simulink model "AdaptiveMPC_Simulation"  (R2020a)
settings: Solver=ode45  StartTime=0  StopTime=150  MaxStep=0.5*Ts  RelTol=1e-3  EnableMultiTasking=on
values from neighbouring files (symbols this model uses):
  Ts = 0.5    [MPC_controller_parameters.m]
  u0 = [op_report.Inputs(1).u;op_report.Inputs(2).u;op_report.Inputs(3).u]    [MPC_controller_parameters.m]
  x0 = [op_report.States(1).x;op_report.States(2).x]    [MPC_controller_parameters.m]
  y0 = [op_report.Outputs(1).y;op_report.Outputs(2).y]    [MPC_controller_parameters.m]
libraries: mpclib x1, dspstat3 x1, slident x1, simulink x1
settings Model: Creator=The MathWorks, Inc.  LastModifiedBy=Mirza
settings DataIOCC: ExternalInput=ExtIn  InitialState=[311.267; 8.5695]  SaveFormat=Structure  SaveOutput=off  SignalLogging=off  DSMLogging=off  SaveTime=off  ReturnWorkspaceOutputs=off  SignalLoggingName=logsOut
settings OptimizationCC: BooleanDataType=off  DefaultParameterBehavior=Inlined  InlineInvariantSignals=on  BufferReuse=off  ExpressionDepthLimit=2147483647  InitFltsAndDblsToZero=on  LifeSpan=inf
settings DebuggingCC: SaveWithParameterizedLinksMsg=none  UnderspecifiedInitializationDetection=Classic  MergeDetectMultiDrivingBlocksExec=none  CheckExecutionContextPreStartOutputMsg=on  CheckExecutionContextRuntimeOutputMsg=on  SignalResolutionControl=TryResolveAllWithWarning  MultiTaskDSMMsg=warning  MultiTaskCondExecSysMsg=none  StateNameClashWarn=warning  SFUnexpectedBacktrackingDiag=warning  SFNoUnconditionalDefaultTransitionDiag=warning  SFExecutionAtInitializationDiag=none  ArithmeticOperatorsInVariantConditions=warning
settings HardwareCC: ProdBitPerPointer=32  ProdBitPerSizeT=32  ProdBitPerPtrDiffT=32  ProdLargestAtomicFloat=None  ProdIntDivRoundTo=Undefined  ProdEndianess=Unspecified  ProdWordSize=32  ProdHWDeviceType=32-bit Generic  TargetUnknown=on
settings ModelReferenceCC: PropagateSignalLabelsOutOfModel=off
settings SFSimCC: SimUseLocalCustomCode=off  CustomCodeUndefinedFunction=UseInterfaceOnly
settings RTWCC: RTWUseLocalCustomCode=off
settings CodeAppCC: StateflowObjectComments=on
settings GRTTargetCC: TargetFcnLib=ansi_tfl_tmw.mat  TargetLangStandard=C89/C90 (ANSI)  CombineOutputUpdateFcns=off  GRTInterface=on
settings ConfigComp: CovMetricSettings=dw  CovHtmlReporting=on  CovSaveCumulativeToWorkspaceVar=on  CovSaveSingleToWorkspaceVar=on  CovExternalEMLEnable=off  CovSFcnEnable=off

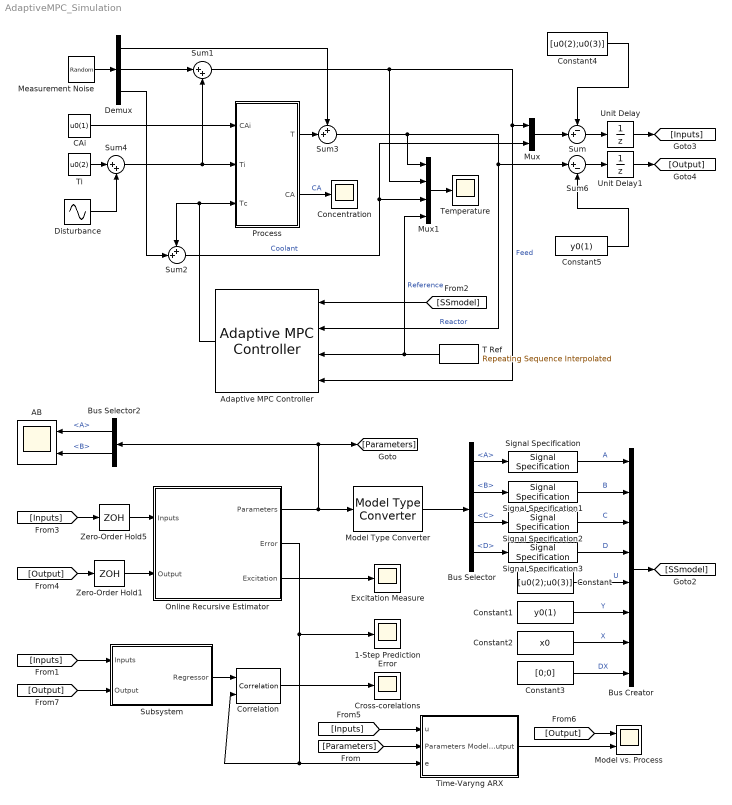
== system AdaptiveMPC_Simulation ==
  1-Step Prediction Error : Scope
  AB : Scope  NumInputPorts=2
  Adaptive MPC Controller : mpclib/Adaptive MPC Controller  SCDEnableBlockLinearizationSpecification=on  mpcobj=mpcobj  enable_value=0  updateMPCinCallerWorkspace=on  md_inport=on  mv_inport=off  uref_inport=off  return_cost=off  return_mvseq=off  return_qpstatus=off  return_xseq=off  return_state=off  return_ovseq=off  state_inport=off  isltv_plant=off  umin_inport=off  umax_inport=off  ymin_inport=off  ymax_inport=off  cc_inport=off  ywt_inport=off  uwt_inport=off  duwt_inport=off  rhoeps_inport=off  pm_inport=off  MaximumP=10  HorizonChoice=FixedHorizon  BlockDataType=double  SampleTimeInherited=off  switch_inport=off
  Bus Creator : BusCreator  Inputs=8
  Bus Selector : BusSelector  OutputSignals=A,B,C,D
  Bus Selector2 : BusSelector  OutputSignals=A,B
  CAi : Constant  Value=u0(1)
  Concentration : Scope
  Constant : Constant  Value=[u0(2);u0(3)]  VectorParams1D=off
  Constant1 : Constant  Value=y0(1)  VectorParams1D=off
  Constant2 : Constant  Value=x0  VectorParams1D=off
  Constant3 : Constant  Value=[0;0]  VectorParams1D=off
  Constant4 : Constant  Value=[u0(2);u0(3)]
  Constant5 : Constant  Value=y0(1)
  Correlation : dspstat3/Correlation  domain=Time  roundingMode=Floor  overflowMode=off  outputDataTypeStr=Inherit: Same as accumulator  outputMin=[]  outputMax=[]  outputLastDataTypeStr=Inherit: Same as accumulator
      settings: SourceProductBaseCode=DS
  Cross-corelations : Scope
  Demux : Demux  Outputs=3
  Disturbance : Sin  Amplitude=5  Frequency=0.05  SampleTime=0
  Excitation Measure : Scope
  Measurement Noise : RandomNumber  Mean=[0 0 0]  Variance=0.001*[1 1 1]  Seed=12345  SampleTime=Ts/5
  Model Type Converter : slident/Estimators/Model Type Converter  InputModelType=ARX
      settings: SourceProductBaseCode=ID
  Model vs. Process : Scope  NumInputPorts=2
  Mux : Mux  Inputs=2
  Mux1 : Mux
  Online Recursive Estimator : Subsystem  mask{ModelStructure=ARX, A0=2, B0=[2 2], F0=2, C0=2, D0=2, d=[0 0], P0=10, History=Infinitna, WindowLength=100, EstimationMethod=Kalmanov filter, Lambda=1 - 5e-3, ProcessNoiseCovariance=1, Tolerance=0.0001, AddEnablePort=off, EstimationError=on, ExcitationMeasure=on, SampleTime=0.5}
      mask prompts: ModelStructure "Izbor modela:"; A0 "Broj parametara u A(q) (na):"; B0 "Broj parametara u B(q) (nb):"; F0 "Broj parametara u F(q) (nf):"; C0 "Broj parametara u C(q) (nc):"; D0 "Broj parametara u D(q) (nd):"; d "Kasnjenje ulaza (nk):"; P0 "Matrica kovarijanse parametara:"; History "Historija:"; WindowLength "Sirina prozora:"; EstimationMethod "Metod estimacije:"; Lambda "Faktor iscezavanja:"; ProcessNoiseCovariance "Kovarijansa procesnog suma:"; Tolerance "Toleranca:"; AddEnablePort "Enable port"; EstimationError "Greska estimacije:"; ExcitationMeasure "Mjera pobude:"; SampleTime "Period uzorkovanja:"
      mask TypeOptions ModelStructure: ARX | ARMAX | BJ | OE
      mask Callback ModelStructure:
      | maskStr = get_param(gcb, 'ModelStructure');
      | maskStr1 = get_param(gcb, 'History');
      | maskStr2 = get_param(gcb, 'EstimationMethod');
      | 
      | if strcmp(maskStr, 'ARX') && strcmp(maskStr1, 'Infinitna') && strcmp(maskStr2, 'Faktor iscezavanja') ,
      |     set_param(gcb, 'MaskVisibilities', {'on';'on';'on';'off';'off';'off';'on';'on';'on';'off';'on';'on';'off';'off';'on';'on';'on';'on'}),
      | elseif strcmp(maskStr, 'ARX') && strcmp(maskStr1, 'Infinitna') && strcmp(maskStr2, 'BFGS') ,
      |     set_param(gcb, 'MaskVisibilities', {'on';'on';'on';'off';'off';'off';'on';'on';'on';'on';'on';'off';'off';'on';'on';'on';'on';'on'}),
      | elseif strcmp(maskStr, 'ARX') && strcmp(maskStr1, 'Infinitna') && strcmp(maskStr2, 'Kalmanov filter') ,
      |     set_param(gcb, 'MaskVisibilities', {'on';'on';'on';'off';'off';'off';'on';'on';'on';'off';'on';'off';'on';'off';'on';'on';'on';'on'}),
      | elseif strcmp(maskStr, 'ARX') && strcmp(maskStr1, 'Finitna') && strcmp(maskStr2, 'Faktor iscezavanja') ,
      |     set_param(gcb, 'MaskVisibilities', {'on';'on';'on';'off';'off';'off';'on';'on';'on';'on';'on';'off';'off';'off';'on';'on';'on';'on'}),
      | elseif strcmp(maskStr, 'ARX') && strcmp(maskStr1, 'Finitna') && strcmp(maskStr2, 'BFGS') ,
      |     set_param(gcb, 'MaskVisibilities', {'on';'on';'on';'off';'off';'off';'on';'on';'on';'on';'on';'off';'off';'on';'on';'on';'on';'on'}),
      | elseif strcmp(maskStr, 'ARX') && strcmp(maskStr1, 'Finitna') && strcmp(maskStr2, 'Kalmanov filter') ,
      |     set_param(gcb, 'MaskVisibilities', {'on';'on';'on';'off';'off';'off';'on';'on';'on';'on';'on';'off';'off';'off';'on';'on';'on';'on'}),
      | elseif strcmp(maskStr, 'ARMAX') && strcmp(maskStr1, 'Infinitna') && strcmp(maskStr2, 'Faktor iscezavanja') ,
      |     set_param(gcb, 'MaskVisibilities', {'on';'on';'on';'off';'on';'off';'on';'on';'on';'off';'on';'on';'off';'off';'on';'on';'on';'on'}),
      | elseif strcmp(maskStr, 'ARMAX') && strcmp(maskStr1, 'Infinitna') && strcmp(maskStr2, 'BFGS') ,
      |     set_param(gcb, 'MaskVisibilities', {'on';'on';'on';'off';'on';'off';'on';'on';'on';'on';'on';'off';'off';'on';'on';'on';'on';'on'}),
      | elseif strcmp(maskStr, 'ARMAX') && strcmp(maskStr1, 'Infinitna') && strcmp(maskStr2, 'Kalmanov filter') ,
      |     set_param(gcb, 'MaskVisibilities', {'on';'on';'on';'off';'on';'off';'on';'on';'on';'off';'on';'off';'on';'off';'on';'on';'on';'on'}),
      | elseif strcmp(maskStr, 'ARMAX') && strcmp(maskStr1, 'Finitna') && strcmp(maskStr2, 'Faktor iscezavanja') ,
      |     set_param(gcb, 'MaskVisibilities', {'on';'on';'on';'off';'on';'off';'on';'on';'on';'on';'on';'off';'off';'off';'on';'on';'on';'on'}),
      | elseif strcmp(maskStr, 'ARMAX') && strcmp(maskStr1, 'Finitna') && strcmp(maskStr2, 'BFGS') ,
      |     set_param(gcb, 'MaskVisibilities', {'on';'on';'on';'off';'on';'off';'on';'on';'on';'on';'on';'off';'off';'on';'on';'on';'on';'on'}),
      | elseif strcmp(maskStr, 'ARMAX') && strcmp(maskStr1, 'Finitna') && strcmp(maskStr2, 'Kalmanov filter') ,
      |     set_param(gcb, 'MaskVisibilities', {'on';'on';'on';'off';'on';'off';'on';'on';'on';'on';'on';'off';'off';'off';'on';'on';'on';'on'}),
      | elseif strcmp(maskStr, 'BJ') && strcmp(maskStr1, 'Infinitna') && strcmp(maskStr2, 'Faktor iscezavanja') ,
      |     set_param(gcb, 'MaskVisibilities', {'on';'off';'on';'on';'on';'on';'on';'on';'on';'off';'on';'on';'off';'off';'on';'on';'on';'on'}),
      | elseif strcmp(maskStr, 'BJ') && strcmp(maskStr1, 'Infinitna') && strcmp(maskStr2, 'BFGS') ,
      |     set_param(gcb, 'MaskVisibilities', {'on';'off';'on';'on';'on';'on';'on';'on';'on';'on';'on';'off';'off';'on';'on';'on';'on';'on'}),
      | elseif strcmp(maskStr, 'BJ') && strcmp(maskStr1, 'Infinitna') && strcmp(maskStr2, 'Kalmanov filter') ,
      |     set_param(gcb, 'MaskVisibilities', {'on';'off';'on';'on';'on';'on';'on';'on';'on';'off';'on';'off';'on';'off';'on';'on';'on';'on'}),
      | elseif strcmp(maskStr, 'BJ') && strcmp(maskStr1, 'Finitna') && strcmp(maskStr2, 'Faktor iscezavanja') ,
      |     set_param(gcb, 'MaskVisibilities', {'on';'off';'on';'on';'on';'on';'on';'on';'on';'on';'on';'off';'off';'off';'on';'on';'on';'on'}),
      | elseif strcmp(maskStr, 'BJ') && strcmp(maskStr1, 'Finitna') && strcmp(maskStr2, 'BFGS') ,
      |     set_param(gcb, 'MaskVisibilities', {'on';'off';'on';'on';'on';'on';'on';'on';'on';'on';'on';'off';'off';'on';'on';'on';'on';'on'}),
      | elseif strcmp(maskStr, 'BJ') && strcmp(maskStr1, 'Finitna') && strcmp(maskStr2, 'Kalmanov filter') ,
      |     set_param(gcb, 'MaskVisibilities', {'on';'off';'on';'on';'on';'on';'on';'on';'on';'on';'on';'off';'off';'off';'on';'on';'on';'on'}),
      | elseif strcmp(maskStr, 'OE') && strcmp(maskStr1, 'Infinitna') && strcmp(maskStr2, 'Faktor iscezavanja') ,
      |     set_param(gcb, 'MaskVisibilities', {'on';'off';'on';'on';'off';'off';'on';'on';'on';'off';'on';'on';'off';'off';'on';'on';'on';'on'}),
      | elseif strcmp(maskStr, 'OE') && strcmp(maskStr1, 'Infinitna') && strcmp(maskStr2, 'BFGS') ,
      |     set_param(gcb, 'MaskVisibilities', {'on';'off';'on';'on';'off';'off';'on';'on';'on';'on';'on';'off';'off';'on';'on';'on';'on';'on'}),
      | elseif strcmp(maskStr, 'OE') && strcmp(maskStr1, 'Infinitna') && strcmp(maskStr2, 'Kalmanov filter') ,
      |     set_param(gcb, 'MaskVisibilities', {'on';'off';'on';'on';'off';'off';'on';'on';'on';'off';'on';'off';'on';'off';'on';'on';'on';'on'}),
      | elseif strcmp(maskStr, 'OE') && strcmp(maskStr1, 'Finitna') && strcmp(maskStr2, 'Faktor iscezavanja') ,
      |     set_param(gcb, 'MaskVisibilities', {'on';'off';'on';'on';'off';'off';'on';'on';'on';'on';'on';'off';'off';'off';'on';'on';'on';'on'}),
      | elseif strcmp(maskStr, 'OE') && strcmp(maskStr1, 'Finitna') && strcmp(maskStr2, 'BFGS') ,
      |     set_param(gcb, 'MaskVisibilities', {'on';'off';'on';'on';'off';'off';'on';'on';'on';'on';'on';'off';'off';'on';'on';'on';'on';'on'}),
      | elseif strcmp(maskStr, 'OE') && strcmp(maskStr1, 'Finitna') && strcmp(maskStr2, 'Kalmanov filter') ,
      |     set_param(gcb, 'MaskVisibilities', {'on';'off';'on';'on';'off';'off';'on';'on';'on';'on';'on';'off';'off';'off';'on';'on';'on';'on'}),
      | end
      mask TypeOptions History: Infinitna | Finitna
      mask Callback History:
      | maskStr = get_param(gcb, 'ModelStructure');
      | maskStr1 = get_param(gcb, 'History');
      | maskStr2 = get_param(gcb, 'EstimationMethod');
      | 
      | if strcmp(maskStr, 'ARX') && strcmp(maskStr1, 'Infinitna') && strcmp(maskStr2, 'Faktor iscezavanja') ,
      |     set_param(gcb, 'MaskVisibilities', {'on';'on';'on';'off';'off';'off';'on';'on';'on';'off';'on';'on';'off';'off';'on';'on';'on';'on'}),
      | elseif strcmp(maskStr, 'ARX') && strcmp(maskStr1, 'Infinitna') && strcmp(maskStr2, 'BFGS') ,
      |     set_param(gcb, 'MaskVisibilities', {'on';'on';'on';'off';'off';'off';'on';'on';'on';'on';'on';'off';'off';'on';'on';'on';'on';'on'}),
      | elseif strcmp(maskStr, 'ARX') && strcmp(maskStr1, 'Infinitna') && strcmp(maskStr2, 'Kalmanov filter') ,
      |     set_param(gcb, 'MaskVisibilities', {'on';'on';'on';'off';'off';'off';'on';'on';'on';'off';'on';'off';'on';'off';'on';'on';'on';'on'}),
      | elseif strcmp(maskStr, 'ARX') && strcmp(maskStr1, 'Finitna') && strcmp(maskStr2, 'Faktor iscezavanja') ,
      |     set_param(gcb, 'MaskVisibilities', {'on';'on';'on';'off';'off';'off';'on';'on';'on';'on';'on';'off';'off';'off';'on';'on';'on';'on'}),
      | elseif strcmp(maskStr, 'ARX') && strcmp(maskStr1, 'Finitna') && strcmp(maskStr2, 'BFGS') ,
      |     set_param(gcb, 'MaskVisibilities', {'on';'on';'on';'off';'off';'off';'on';'on';'on';'on';'on';'off';'off';'on';'on';'on';'on';'on'}),
      | elseif strcmp(maskStr, 'ARX') && strcmp(maskStr1, 'Finitna') && strcmp(maskStr2, 'Kalmanov filter') ,
      |     set_param(gcb, 'MaskVisibilities', {'on';'on';'on';'off';'off';'off';'on';'on';'on';'on';'on';'off';'off';'off';'on';'on';'on';'on'}),
      | elseif strcmp(maskStr, 'ARMAX') && strcmp(maskStr1, 'Infinitna') && strcmp(maskStr2, 'Faktor iscezavanja') ,
      |     set_param(gcb, 'MaskVisibilities', {'on';'on';'on';'off';'on';'off';'on';'on';'on';'off';'on';'on';'off';'off';'on';'on';'on';'on'}),
      | elseif strcmp(maskStr, 'ARMAX') && strcmp(maskStr1, 'Infinitna') && strcmp(maskStr2, 'BFGS') ,
      |     set_param(gcb, 'MaskVisibilities', {'on';'on';'on';'off';'on';'off';'on';'on';'on';'on';'on';'off';'off';'on';'on';'on';'on';'on'}),
      | elseif strcmp(maskStr, 'ARMAX') && strcmp(maskStr1, 'Infinitna') && strcmp(maskStr2, 'Kalmanov filter') ,
      |     set_param(gcb, 'MaskVisibilities', {'on';'on';'on';'off';'on';'off';'on';'on';'on';'off';'on';'off';'on';'off';'on';'on';'on';'on'}),
      | elseif strcmp(maskStr, 'ARMAX') && strcmp(maskStr1, 'Finitna') && strcmp(maskStr2, 'Faktor iscezavanja') ,
      |     set_param(gcb, 'MaskVisibilities', {'on';'on';'on';'off';'on';'off';'on';'on';'on';'on';'on';'off';'off';'off';'on';'on';'on';'on'}),
      | elseif strcmp(maskStr, 'ARMAX') && strcmp(maskStr1, 'Finitna') && strcmp(maskStr2, 'BFGS') ,
      |     set_param(gcb, 'MaskVisibilities', {'on';'on';'on';'off';'on';'off';'on';'on';'on';'on';'on';'off';'off';'on';'on';'on';'on';'on'}),
      | elseif strcmp(maskStr, 'ARMAX') && strcmp(maskStr1, 'Finitna') && strcmp(maskStr2, 'Kalmanov filter') ,
      |     set_param(gcb, 'MaskVisibilities', {'on';'on';'on';'off';'on';'off';'on';'on';'on';'on';'on';'off';'off';'off';'on';'on';'on';'on'}),
      | elseif strcmp(maskStr, 'BJ') && strcmp(maskStr1, 'Infinitna') && strcmp(maskStr2, 'Faktor iscezavanja') ,
      |     set_param(gcb, 'MaskVisibilities', {'on';'off';'on';'on';'on';'on';'on';'on';'on';'off';'on';'on';'off';'off';'on';'on';'on';'on'}),
      | elseif strcmp(maskStr, 'BJ') && strcmp(maskStr1, 'Infinitna') && strcmp(maskStr2, 'BFGS') ,
      |     set_param(gcb, 'MaskVisibilities', {'on';'off';'on';'on';'on';'on';'on';'on';'on';'on';'on';'off';'off';'on';'on';'on';'on';'on'}),
      | elseif strcmp(maskStr, 'BJ') && strcmp(maskStr1, 'Infinitna') && strcmp(maskStr2, 'Kalmanov filter') ,
      |     set_param(gcb, 'MaskVisibilities', {'on';'off';'on';'on';'on';'on';'on';'on';'on';'off';'on';'off';'on';'off';'on';'on';'on';'on'}),
      | elseif strcmp(maskStr, 'BJ') && strcmp(maskStr1, 'Finitna') && strcmp(maskStr2, 'Faktor iscezavanja') ,
      |     set_param(gcb, 'MaskVisibilities', {'on';'off';'on';'on';'on';'on';'on';'on';'on';'on';'on';'off';'off';'off';'on';'on';'on';'on'}),
      | elseif strcmp(maskStr, 'BJ') && strcmp(maskStr1, 'Finitna') && strcmp(maskStr2, 'BFGS') ,
      |     set_param(gcb, 'MaskVisibilities', {'on';'off';'on';'on';'on';'on';'on';'on';'on';'on';'on';'off';'off';'on';'on';'on';'on';'on'}),
      | elseif strcmp(maskStr, 'BJ') && strcmp(maskStr1, 'Finitna') && strcmp(maskStr2, 'Kalmanov filter') ,
      |     set_param(gcb, 'MaskVisibilities', {'on';'off';'on';'on';'on';'on';'on';'on';'on';'on';'on';'off';'off';'off';'on';'on';'on';'on'}),
      | elseif strcmp(maskStr, 'OE') && strcmp(maskStr1, 'Infinitna') && strcmp(maskStr2, 'Faktor iscezavanja') ,
      |     set_param(gcb, 'MaskVisibilities', {'on';'off';'on';'on';'off';'off';'on';'on';'on';'off';'on';'on';'off';'off';'on';'on';'on';'on'}),
      | elseif strcmp(maskStr, 'OE') && strcmp(maskStr1, 'Infinitna') && strcmp(maskStr2, 'BFGS') ,
      |     set_param(gcb, 'MaskVisibilities', {'on';'off';'on';'on';'off';'off';'on';'on';'on';'on';'on';'off';'off';'on';'on';'on';'on';'on'}),
      | elseif strcmp(maskStr, 'OE') && strcmp(maskStr1, 'Infinitna') && strcmp(maskStr2, 'Kalmanov filter') ,
      |     set_param(gcb, 'MaskVisibilities', {'on';'off';'on';'on';'off';'off';'on';'on';'on';'off';'on';'off';'on';'off';'on';'on';'on';'on'}),
      | elseif strcmp(maskStr, 'OE') && strcmp(maskStr1, 'Finitna') && strcmp(maskStr2, 'Faktor iscezavanja') ,
      |     set_param(gcb, 'MaskVisibilities', {'on';'off';'on';'on';'off';'off';'on';'on';'on';'on';'on';'off';'off';'off';'on';'on';'on';'on'}),
      | elseif strcmp(maskStr, 'OE') && strcmp(maskStr1, 'Finitna') && strcmp(maskStr2, 'BFGS') ,
      |     set_param(gcb, 'MaskVisibilities', {'on';'off';'on';'on';'off';'off';'on';'on';'on';'on';'on';'off';'off';'on';'on';'on';'on';'on'}),
      | elseif strcmp(maskStr, 'OE') && strcmp(maskStr1, 'Finitna') && strcmp(maskStr2, 'Kalmanov filter') ,
      |     set_param(gcb, 'MaskVisibilities', {'on';'off';'on';'on';'off';'off';'on';'on';'on';'on';'on';'off';'off';'off';'on';'on';'on';'on'}),
      | end
      mask TypeOptions EstimationMethod: Faktor iscezavanja | BFGS | Kalmanov filter
      mask Callback EstimationMethod:
      | maskStr = get_param(gcb, 'ModelStructure');
      | maskStr1 = get_param(gcb, 'History');
      | maskStr2 = get_param(gcb, 'EstimationMethod');
      | 
      | if strcmp(maskStr, 'ARX') && strcmp(maskStr1, 'Infinitna') && strcmp(maskStr2, 'Faktor iscezavanja') ,
      |     set_param(gcb, 'MaskVisibilities', {'on';'on';'on';'off';'off';'off';'on';'on';'on';'off';'on';'on';'off';'off';'on';'on';'on';'on'}),
      | elseif strcmp(maskStr, 'ARX') && strcmp(maskStr1, 'Infinitna') && strcmp(maskStr2, 'BFGS') ,
      |     set_param(gcb, 'MaskVisibilities', {'on';'on';'on';'off';'off';'off';'on';'on';'on';'on';'on';'off';'off';'on';'on';'on';'on';'on'}),
      | elseif strcmp(maskStr, 'ARX') && strcmp(maskStr1, 'Infinitna') && strcmp(maskStr2, 'Kalmanov filter') ,
      |     set_param(gcb, 'MaskVisibilities', {'on';'on';'on';'off';'off';'off';'on';'on';'on';'off';'on';'off';'on';'off';'on';'on';'on';'on'}),
      | elseif strcmp(maskStr, 'ARX') && strcmp(maskStr1, 'Finitna') && strcmp(maskStr2, 'Faktor iscezavanja') ,
      |     set_param(gcb, 'MaskVisibilities', {'on';'on';'on';'off';'off';'off';'on';'on';'on';'on';'on';'off';'off';'off';'on';'on';'on';'on'}),
      | elseif strcmp(maskStr, 'ARX') && strcmp(maskStr1, 'Finitna') && strcmp(maskStr2, 'BFGS') ,
      |     set_param(gcb, 'MaskVisibilities', {'on';'on';'on';'off';'off';'off';'on';'on';'on';'on';'on';'off';'off';'on';'on';'on';'on';'on'}),
      | elseif strcmp(maskStr, 'ARX') && strcmp(maskStr1, 'Finitna') && strcmp(maskStr2, 'Kalmanov filter') ,
      |     set_param(gcb, 'MaskVisibilities', {'on';'on';'on';'off';'off';'off';'on';'on';'on';'on';'on';'off';'off';'off';'on';'on';'on';'on'}),
      | elseif strcmp(maskStr, 'ARMAX') && strcmp(maskStr1, 'Infinitna') && strcmp(maskStr2, 'Faktor iscezavanja') ,
      |     set_param(gcb, 'MaskVisibilities', {'on';'on';'on';'off';'on';'off';'on';'on';'on';'off';'on';'on';'off';'off';'on';'on';'on';'on'}),
      | elseif strcmp(maskStr, 'ARMAX') && strcmp(maskStr1, 'Infinitna') && strcmp(maskStr2, 'BFGS') ,
      |     set_param(gcb, 'MaskVisibilities', {'on';'on';'on';'off';'on';'off';'on';'on';'on';'on';'on';'off';'off';'on';'on';'on';'on';'on'}),
      | elseif strcmp(maskStr, 'ARMAX') && strcmp(maskStr1, 'Infinitna') && strcmp(maskStr2, 'Kalmanov filter') ,
      |     set_param(gcb, 'MaskVisibilities', {'on';'on';'on';'off';'on';'off';'on';'on';'on';'off';'on';'off';'on';'off';'on';'on';'on';'on'}),
      | elseif strcmp(maskStr, 'ARMAX') && strcmp(maskStr1, 'Finitna') && strcmp(maskStr2, 'Faktor iscezavanja') ,
      |     set_param(gcb, 'MaskVisibilities', {'on';'on';'on';'off';'on';'off';'on';'on';'on';'on';'on';'off';'off';'off';'on';'on';'on';'on'}),
      | elseif strcmp(maskStr, 'ARMAX') && strcmp(maskStr1, 'Finitna') && strcmp(maskStr2, 'BFGS') ,
      |     set_param(gcb, 'MaskVisibilities', {'on';'on';'on';'off';'on';'off';'on';'on';'on';'on';'on';'off';'off';'on';'on';'on';'on';'on'}),
      | elseif strcmp(maskStr, 'ARMAX') && strcmp(maskStr1, 'Finitna') && strcmp(maskStr2, 'Kalmanov filter') ,
      |     set_param(gcb, 'MaskVisibilities', {'on';'on';'on';'off';'on';'off';'on';'on';'on';'on';'on';'off';'off';'off';'on';'on';'on';'on'}),
      | elseif strcmp(maskStr, 'BJ') && strcmp(maskStr1, 'Infinitna') && strcmp(maskStr2, 'Faktor iscezavanja') ,
      |     set_param(gcb, 'MaskVisibilities', {'on';'off';'on';'on';'on';'on';'on';'on';'on';'off';'on';'on';'off';'off';'on';'on';'on';'on'}),
      | elseif strcmp(maskStr, 'BJ') && strcmp(maskStr1, 'Infinitna') && strcmp(maskStr2, 'BFGS') ,
      |     set_param(gcb, 'MaskVisibilities', {'on';'off';'on';'on';'on';'on';'on';'on';'on';'on';'on';'off';'off';'on';'on';'on';'on';'on'}),
      | elseif strcmp(maskStr, 'BJ') && strcmp(maskStr1, 'Infinitna') && strcmp(maskStr2, 'Kalmanov filter') ,
      |     set_param(gcb, 'MaskVisibilities', {'on';'off';'on';'on';'on';'on';'on';'on';'on';'off';'on';'off';'on';'off';'on';'on';'on';'on'}),
      | elseif strcmp(maskStr, 'BJ') && strcmp(maskStr1, 'Finitna') && strcmp(maskStr2, 'Faktor iscezavanja') ,
      |     set_param(gcb, 'MaskVisibilities', {'on';'off';'on';'on';'on';'on';'on';'on';'on';'on';'on';'off';'off';'off';'on';'on';'on';'on'}),
      | elseif strcmp(maskStr, 'BJ') && strcmp(maskStr1, 'Finitna') && strcmp(maskStr2, 'BFGS') ,
      |     set_param(gcb, 'MaskVisibilities', {'on';'off';'on';'on';'on';'on';'on';'on';'on';'on';'on';'off';'off';'on';'on';'on';'on';'on'}),
      | elseif strcmp(maskStr, 'BJ') && strcmp(maskStr1, 'Finitna') && strcmp(maskStr2, 'Kalmanov filter') ,
      |     set_param(gcb, 'MaskVisibilities', {'on';'off';'on';'on';'on';'on';'on';'on';'on';'on';'on';'off';'off';'off';'on';'on';'on';'on'}),
      | elseif strcmp(maskStr, 'OE') && strcmp(maskStr1, 'Infinitna') && strcmp(maskStr2, 'Faktor iscezavanja') ,
      |     set_param(gcb, 'MaskVisibilities', {'on';'off';'on';'on';'off';'off';'on';'on';'on';'off';'on';'on';'off';'off';'on';'on';'on';'on'}),
      | elseif strcmp(maskStr, 'OE') && strcmp(maskStr1, 'Infinitna') && strcmp(maskStr2, 'BFGS') ,
      |     set_param(gcb, 'MaskVisibilities', {'on';'off';'on';'on';'off';'off';'on';'on';'on';'on';'on';'off';'off';'on';'on';'on';'on';'on'}),
      | elseif strcmp(maskStr, 'OE') && strcmp(maskStr1, 'Infinitna') && strcmp(maskStr2, 'Kalmanov filter') ,
      |     set_param(gcb, 'MaskVisibilities', {'on';'off';'on';'on';'off';'off';'on';'on';'on';'off';'on';'off';'on';'off';'on';'on';'on';'on'}),
      | elseif strcmp(maskStr, 'OE') && strcmp(maskStr1, 'Finitna') && strcmp(maskStr2, 'Faktor iscezavanja') ,
      |     set_param(gcb, 'MaskVisibilities', {'on';'off';'on';'on';'off';'off';'on';'on';'on';'on';'on';'off';'off';'off';'on';'on';'on';'on'}),
      | elseif strcmp(maskStr, 'OE') && strcmp(maskStr1, 'Finitna') && strcmp(maskStr2, 'BFGS') ,
      |     set_param(gcb, 'MaskVisibilities', {'on';'off';'on';'on';'off';'off';'on';'on';'on';'on';'on';'off';'off';'on';'on';'on';'on';'on'}),
      | elseif strcmp(maskStr, 'OE') && strcmp(maskStr1, 'Finitna') && strcmp(maskStr2, 'Kalmanov filter') ,
      |     set_param(gcb, 'MaskVisibilities', {'on';'off';'on';'on';'off';'off';'on';'on';'on';'on';'on';'off';'off';'off';'on';'on';'on';'on'}),
      | end
      mask Callback AddEnablePort:
      | maskStr3 = get_param(gcb, 'AddEnablePort');
      | 
      | if strcmp(maskStr3, 'on')
      |      if (getSimulinkBlockHandle('PSAU_SeminarskiRad_AdaptiveMPC/Online Recursive Estimator/EnableConst')>0)
      |           delete_line('PSAU_SeminarskiRad_AdaptiveMPC/Online Recursive Estimator', 'EnableConst/1', 'Data Type Conversion/1');
      |           delete_block('PSAU_SeminarskiRad_AdaptiveMPC/Online Recursive Estimator/EnableConst');
      |      end
      |      if (getSimulinkBlockHandle('PSAU_SeminarskiRad_AdaptiveMPC/Online Recursive Estimator/Enable')==-1)
      |           add_block('simulink/Sources/In1','PSAU_SeminarskiRad_AdaptiveMPC/Online Recursive Estimator/Enable');
      |           set_param('PSAU_SeminarskiRad_AdaptiveMPC/Online Recursive Estimator/Enable','position',[510, 403, 540, 417]);
      |           add_line('PSAU_SeminarskiRad_AdaptiveMPC/Online Recursive Estimator', 'Enable/1', 'Data Type Conversion/1');
      |      end
      | elseif strcmp(maskStr3, 'off')
      |     if (getSimulinkBlockHandle('PSAU_SeminarskiRad_AdaptiveMPC/Online Recursive Estimator/Enable')>0)
      |          delete_line('PSAU_SeminarskiRad_AdaptiveMPC/Online Recursive Estimator', 'Enable/1', 'Data Type Conversion/1');
      |          delete_block('PSAU_SeminarskiRad_AdaptiveMPC/Online Recursive Estimator/Enable');
      |     end
      |     if (getSimulinkBlockHandle('PSAU_SeminarskiRad_AdaptiveMPC/Online Recursive Estimator/EnableConst')==-1)
      |          add_block('simulink/Sources/Constant','PSAU_SeminarskiRad_AdaptiveMPC/Online Recursive Estimator/EnableConst');
      |          set_param('PSAU_SeminarskiRad_AdaptiveMPC/Online Recursive Estimator/EnableConst','position',[510, 395, 540, 425]);
      |          add_line('PSAU_SeminarskiRad_AdaptiveMPC/Online Recursive Estimator', 'EnableConst/1', 'Data Type Conversion/1');
      |     end
      | end
      mask Callback EstimationError:
      | maskStr4 = get_param(gcb, 'EstimationError');
      | 
      | if strcmp(maskStr4, 'on')
      |      if (getSimulinkBlockHandle('PSAU_SeminarskiRad_AdaptiveMPC/Online Recursive Estimator/ETerminator')>0)
      |           delete_line('PSAU_SeminarskiRad_AdaptiveMPC/Online Recursive Estimator', 'sf/2', 'ETerminator/1');
      |           delete_block('PSAU_SeminarskiRad_AdaptiveMPC/Online Recursive Estimator/ETerminator');
      |      end
      |      if (getSimulinkBlockHandle('PSAU_SeminarskiRad_AdaptiveMPC/Online Recursive Estimator/Error')==-1)
      |           add_block('simulink/Sinks/Out1','PSAU_SeminarskiRad_AdaptiveMPC/Online Recursive Estimator/Error');
      |           set_param('PSAU_SeminarskiRad_AdaptiveMPC/Online Recursive Estimator/Error','position',[1080, 335, 1110, 365]);
      |           add_line('PSAU_SeminarskiRad_AdaptiveMPC/Online Recursive Estimator', 'sf/2', 'Error/1');
      |      end
      | elseif strcmp(maskStr4, 'off')
      |     if (getSimulinkBlockHandle('PSAU_SeminarskiRad_AdaptiveMPC/Online Recursive Estimator/Error')>0)
      |          delete_line('PSAU_SeminarskiRad_AdaptiveMPC/Online Recursive Estimator', 'sf/2', 'Error/1');
      |          delete_block('PSAU_SeminarskiRad_AdaptiveMPC/Online Recursive Estimator/Error');
      |     end
      |     if (getSimulinkBlockHandle('PSAU_SeminarskiRad_AdaptiveMPC/Online Recursive Estimator/ETerminator')==-1)
      |          add_block('simulink/Commonly Used Blocks/Terminator','PSAU_SeminarskiRad_AdaptiveMPC/Online Recursive Estimator/ETerminator');
      |          set_param('PSAU_SeminarskiRad_AdaptiveMPC/Online Recursive Estimator/ETerminator','position',[1080, 335, 1110, 365]);
      |          add_line('PSAU_SeminarskiRad_AdaptiveMPC/Online Recursive Estimator', 'sf/2', 'ETerminator/1');
      |     end
      | end
      mask Callback ExcitationMeasure:
      | maskStr5 = get_param(gcb, 'ExcitationMeasure');
      | 
      | if strcmp(maskStr5, 'on')
      |      if (getSimulinkBlockHandle('PSAU_SeminarskiRad_AdaptiveMPC/Online Recursive Estimator/ExTerminator')>0)
      |           delete_line('PSAU_SeminarskiRad_AdaptiveMPC/Online Recursive Estimator', 'sf/3', 'ExTerminator/1');
      |           delete_block('PSAU_SeminarskiRad_AdaptiveMPC/Online Recursive Estimator/ExTerminator');
      |      end
      |      if (getSimulinkBlockHandle('PSAU_SeminarskiRad_AdaptiveMPC/Online Recursive Estimator/Excitation')==-1)
      |           add_block('simulink/Sinks/Out1','PSAU_SeminarskiRad_AdaptiveMPC/Online Recursive Estimator/Excitation');
      |           set_param('PSAU_SeminarskiRad_AdaptiveMPC/Online Recursive Estimator/Excitation','position',[1080, 403, 1110, 417]);
      |           add_line('PSAU_SeminarskiRad_AdaptiveMPC/Online Recursive Estimator', 'sf/3', 'Excitation/1');
      |      end
      | elseif strcmp(maskStr5, 'off')
      |     if (getSimulinkBlockHandle('PSAU_SeminarskiRad_AdaptiveMPC/Online Recursive Estimator/Excitation')>0)
      |          delete_line('PSAU_SeminarskiRad_AdaptiveMPC/Online Recursive Estimator', 'sf/3', 'Excitation/1');
      |          delete_block('PSAU_SeminarskiRad_AdaptiveMPC/Online Recursive Estimator/Excitation');
      |     end
      |     if (getSimulinkBlockHandle('PSAU_SeminarskiRad_AdaptiveMPC/Online Recursive Estimator/ExTerminator')==-1)
      |          add_block('simulink/Commonly Used Blocks/Terminator','PSAU_SeminarskiRad_AdaptiveMPC/Online Recursive Estimator/ExTerminator');
      |          set_param('PSAU_SeminarskiRad_AdaptiveMPC/Online Recursive Estimator/ExTerminator','position',[1080, 403, 1110, 417]);
      |          add_line('PSAU_SeminarskiRad_AdaptiveMPC/Online Recursive Estimator', 'sf/3', 'ExTerminator/1');
      |     end
      | end
      mask DialogControl DescGroupVar Prompt: Rekurzivna estimacija parametara
      mask DialogControl DescTextVar Prompt: Blok za estimaciju parametara linearnih modela sa ARX, ARMAX, BJ i OE strukturom.
      mask DialogControl ContainerModelParameters Prompt: Parametri modela
      mask DialogControl ContainerModelStructure Prompt: Opis modela
      mask DialogControl ContainerAlgorithmAndBlockOptions Prompt: Opcije bloka i algoritma
      mask DialogControl ContainerAlgorithmOptions Prompt: Opcije algoritma
  Process : Subsystem
  Signal Specification : SignalSpecification  Dimensions=[2 2]
  Signal Specification1 : SignalSpecification  Dimensions=[2 2]
  Signal Specification2 : SignalSpecification  Dimensions=[1 2]
  Signal Specification3 : SignalSpecification  Dimensions=[1 2]
  Subsystem : Subsystem
  Sum : Sum  Inputs=-+|
  Sum1 : Sum  Inputs=|++  SampleTime=Ts/5
  Sum2 : Sum  Inputs=++|  SampleTime=Ts/5
  Sum3 : Sum  Inputs=++|  SampleTime=Ts/5
  Sum4 : Sum  Inputs=|++  SampleTime=Ts/5
  Sum6 : Sum  Inputs=|+-
  T Ref : simulink/Sources/Repeating Sequence Interpolated  OutValues=[y0(1) y0(1) 373 373]  TimeValues=[0 50 100 500]  LookUpMeth=Interpolation-Use End Values  tsamp=Ts  OutMin=[]  OutMax=[]  OutDataTypeStr=double  OutputDataTypeScalingMode=double  OutDataType=fixdt(0,8)  OutScaling=2^-10
  Temperature : Scope
  Ti : Constant  Value=u0(2)
  "Time-Varyng ARX " : Subsystem
  Unit Delay : UnitDelay  InitialCondition=[0;0]  SampleTime=Ts  HasFrameUpgradeWarning=on
  Unit Delay1 : UnitDelay  SampleTime=Ts  HasFrameUpgradeWarning=on
  Zero-Order Hold1 : ZeroOrderHold  SampleTime=Ts
  Zero-Order Hold5 : ZeroOrderHold  SampleTime=Ts
  wires:
  Mux1/1 -> Temperature/1
  Sum1/1 -> Adaptive MPC Controller/4, Mux/1, Mux1/2  "Feed"
  Sum2/1 -> Mux/2, Mux1/3  "Coolant"
  Sum3/1 -> Adaptive MPC Controller/2, Sum6/1, Mux1/1  "Reactor"
  Process/2(CA) -> Concentration/1  "CA"
  Process/1(T) -> Sum3/2
  Ti/1 -> Sum4/1
  Sum4/1 -> Sum1/2, Process/2(Ti)
  T Ref/1 -> Adaptive MPC Controller/3, Mux1/4  "Reference"
  Disturbance/1 -> Sum4/2
  Demux/2 -> Sum1/1
  Demux/1 -> Sum3/1
  Demux/3 -> Sum2/2
  Measurement Noise/1 -> Demux/1
  Unit Delay1/1 -> [Output]
  Model Type Converter/1 -> Bus Selector/1
  Constant1/1 -> Bus Creator/6  "Y"
  Constant/1 -> Bus Creator/5  "U"
  Bus Selector/1 -> Signal Specification/1  "<A>"
  Signal Specification/1 -> Bus Creator/1  "A"
  Bus Selector/2 -> Signal Specification1/1  "<B>"
  Bus Selector/3 -> Signal Specification2/1  "<C>"
  Bus Selector/4 -> Signal Specification3/1  "<D>"
  Signal Specification1/1 -> Bus Creator/2  "B"
  Signal Specification2/1 -> Bus Creator/3  "C"
  Signal Specification3/1 -> Bus Creator/4  "D"
  Constant2/1 -> Bus Creator/7  "X"
  Constant3/1 -> Bus Creator/8  "DX"
  Adaptive MPC Controller/1 -> Sum2/1, Process/3(Tc)
  Sum6/1 -> Unit Delay1/1
  Sum/1 -> Unit Delay/1
  Mux/1 -> Sum/2
  Constant4/1 -> Sum/1
  Unit Delay/1 -> [Inputs]
  Constant5/1 -> Sum6/2
  CAi/1 -> Process/1(CAi)
  Bus Selector2/2 -> AB/2  "<B>"
  Bus Selector2/1 -> AB/1  "<A>"
  [Parameters] -> "Time-Varyng ARX "/2(Parameters)
  Zero-Order Hold5/1 -> Online Recursive Estimator/1(Inputs)
  Zero-Order Hold1/1 -> Online Recursive Estimator/2(Output)
  Online Recursive Estimator/1(Parameters) -> Bus Selector2/1, [Parameters], Model Type Converter/1
  Online Recursive Estimator/2(Error) -> Correlation/2, "Time-Varyng ARX "/3(e), 1-Step Prediction Error/1
  Online Recursive Estimator/3(Excitation) -> Excitation Measure/1
  Bus Creator/1 -> [SSmodel]
  [SSmodel] -> Adaptive MPC Controller/1
  "Time-Varyng ARX "/1(Model Output) -> Model vs. Process/2
  [Inputs] -> Zero-Order Hold5/1
  [Output] -> Zero-Order Hold1/1
  [Inputs] -> "Time-Varyng ARX "/1(u)
  [Output] -> Model vs. Process/1
  [Inputs] -> Subsystem/1(Inputs)
  [Output] -> Subsystem/2(Output)
  Subsystem/1(Regressor) -> Correlation/1
  Correlation/1 -> Cross-corelations/1

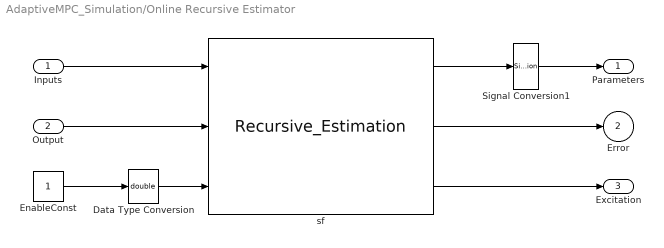
== system AdaptiveMPC_Simulation/Online Recursive Estimator ==
  Inputs : Inport
  Output : Inport  Port=2
  Data Type Conversion : DataTypeConversion  OutDataTypeStr=double
  EnableConst : Constant
  Signal Conversion1 : SignalConversion  ConversionOutput=Virtual bus  OverrideOpt=off
  sf : S-Function  InitFcn=try, set_param(gcb,'FunctionName','Recursive_Estimation'), end  FunctionName=Recursive_Estimation  Parameters=int32(2),int32([2 2]),int32(2),int32(2),int32(0),int32([0 0]),1 - 5e-3,10,int32(1),int32(3),int32(500),0.001,0.1,int32(1),1  SFunctionModules=Recursive_Estimation_wrapper  SFunctionDeploymentMode=off  EnableBusSupport=off  mask(S-Function Builder){}
      mask help: Simulink:masks:SFunctionBuilder_MD
      mask init:
      | val = [[.9  0.75 0.75 1 1 .9 .9 1]',[1 1 0.75 0.75 .9 .9 1 .9]'];try , sys = get_param(gcb,'SfunBuilderFcnName');if isempty(sys), sys = get_param(gcb,'FunctionName'); end,catch, sys = get_param(gcb,'FunctionName'); end
      settings: CopyFcn=set_param(gcbh,'LinkStatus','none')  PreSaveFcn=try, set_param(gcb,'FunctionName','Recursive_Estimation'), end  OpenFcn=sfunctionwizard(gcbh)
      mask Display: plot(val(:,1),val(:,2)),disp(sys), port_label('input',1,'u0'), port_label('input',2,'y0'), port_label('input',3,'Enable'), port_label('output',1,'Params'), port_label('output',2,'Error'), port_label('output',3,'Excitation')
  Parameters : Outport
  Error : Outport  Port=2
  Excitation : Outport  Port=3
  wires:
  sf/1 -> Signal Conversion1/1
  Data Type Conversion/1 -> sf/3
  Signal Conversion1/1 -> Parameters/1
  Output/1 -> sf/2
  Inputs/1 -> sf/1
  sf/2 -> Error/1
  sf/3 -> Excitation/1
  EnableConst/1 -> Data Type Conversion/1

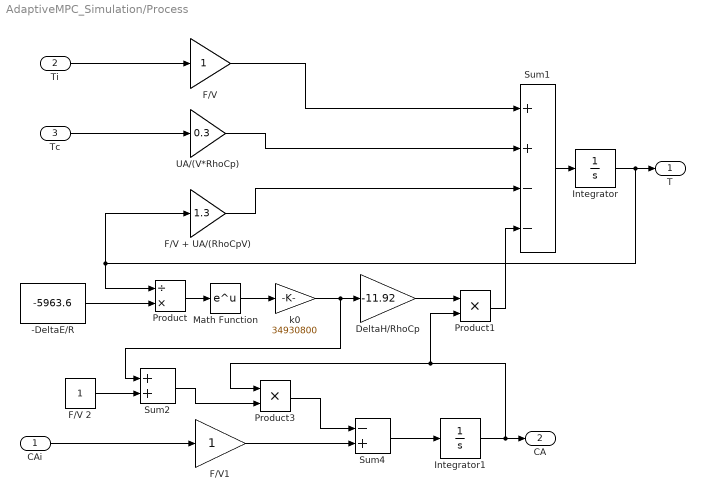
== system AdaptiveMPC_Simulation/Process ==
  CAi : Inport
  Ti : Inport  Port=2
  Tc : Inport  Port=3
  -DeltaE/R : Constant  Value=-5963.6
  DeltaH/RhoCp : Gain  Gain=-11.92  SaturateOnIntegerOverflow=on  OutDataTypeStr=Inherit: Same as input  ParamDataTypeStr=Inherit: Same as input
  F/V : Gain  SaturateOnIntegerOverflow=on  OutDataTypeStr=Inherit: Same as input  ParamDataTypeStr=Inherit: Same as input
  F/V + UA/(RhoCpV) : Gain  Gain=1.3  SaturateOnIntegerOverflow=on  OutDataTypeStr=Inherit: Same as input  ParamDataTypeStr=Inherit: Same as input
  F/V 2 : Constant
  F/V1 : Gain  SaturateOnIntegerOverflow=on  OutDataTypeStr=Inherit: Same as input  ParamDataTypeStr=Inherit: Same as input
  Integrator : Integrator  InitialCondition=311.2639  LimitOutput=on  LowerSaturationLimit=0
  Integrator1 : Integrator  InitialCondition=8.5698  LimitOutput=on  LowerSaturationLimit=0
  Math Function : Math  SignedPower=on  SaturateOnIntegerOverflow=on
  Product : Product  Inputs=/*  InputSameDT=on  RndMeth=Zero  SaturateOnIntegerOverflow=on  OutDataTypeStr=Inherit: Same as first input
  Product1 : Product  InputSameDT=on  RndMeth=Zero  SaturateOnIntegerOverflow=on  OutDataTypeStr=Inherit: Same as first input
  Product3 : Product  InputSameDT=on  RndMeth=Zero  SaturateOnIntegerOverflow=on  OutDataTypeStr=Inherit: Same as first input
  Sum1 : Sum  Inputs=++--  InputSameDT=on  SaturateOnIntegerOverflow=on  OutDataTypeStr=Inherit: Same as first input
  Sum2 : Sum  InputSameDT=on  SaturateOnIntegerOverflow=on  OutDataTypeStr=Inherit: Same as first input
  Sum4 : Sum  Inputs=-+  InputSameDT=on  SaturateOnIntegerOverflow=on  OutDataTypeStr=Inherit: Same as first input
  UA/(V*RhoCp) : Gain  Gain=0.3  SaturateOnIntegerOverflow=on  OutDataTypeStr=Inherit: Same as input  ParamDataTypeStr=Inherit: Same as input
  k0 : Gain  Gain=34930800  SaturateOnIntegerOverflow=on  OutDataTypeStr=Inherit: Same as input  ParamDataTypeStr=Inherit: Same as input
  T : Outport  VectorParamsAs1DForOutWhenUnconnected=off
  CA : Outport  Port=2  VectorParamsAs1DForOutWhenUnconnected=off
  wires:
  Sum2/1 -> Product3/2
  Tc/1 -> UA/(V*RhoCp)/1
  CAi/1 -> F/V1/1
  Ti/1 -> F/V/1
  F/V1/1 -> Sum4/2
  F/V 2/1 -> Sum2/2
  Integrator1/1 -> CA/1, Product3/1, Product1/2
  Sum4/1 -> Integrator1/1
  Product3/1 -> Sum4/1
  -DeltaE/R/1 -> Product/2
  k0/1 -> Sum2/1, DeltaH/RhoCp/1
  Product1/1 -> Sum1/4
  DeltaH/RhoCp/1 -> Product1/1
  Math Function/1 -> k0/1
  Product/1 -> Math Function/1
  F/V + UA/(RhoCpV)/1 -> Sum1/3
  UA/(V*RhoCp)/1 -> Sum1/2
  Integrator/1 -> T/1, F/V + UA/(RhoCpV)/1, Product/1
  Sum1/1 -> Integrator/1
  F/V/1 -> Sum1/1

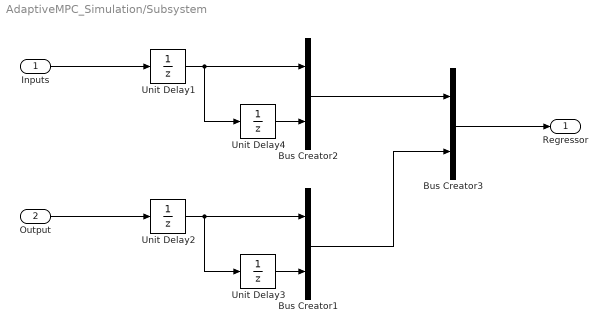
== system AdaptiveMPC_Simulation/Subsystem ==
  Inputs : Inport
  Output : Inport  Port=2
  Bus Creator1 : BusCreator  Inputs=2
  Bus Creator2 : BusCreator  Inputs=2
  Bus Creator3 : BusCreator  Inputs=2
  Unit Delay{1..4} (4 alike) : UnitDelay  SampleTime=-1  HasFrameUpgradeWarning=on
  Regressor : Outport
  wires:
  Unit Delay2/1 -> Unit Delay3/1, Bus Creator1/1
  Unit Delay3/1 -> Bus Creator1/2
  Output/1 -> Unit Delay2/1
  Inputs/1 -> Unit Delay1/1
  Unit Delay1/1 -> Unit Delay4/1, Bus Creator2/1
  Unit Delay4/1 -> Bus Creator2/2
  Bus Creator3/1 -> Regressor/1
  Bus Creator2/1 -> Bus Creator3/1
  Bus Creator1/1 -> Bus Creator3/2

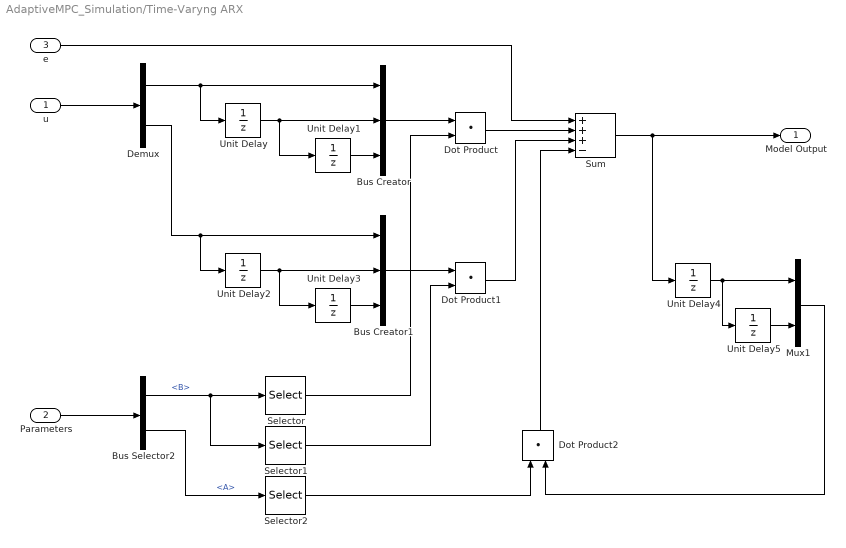
== system AdaptiveMPC_Simulation/Time-Varyng ARX  ==
  u : Inport
  Parameters : Inport  Port=2
  e : Inport  Port=3
  Bus Creator : BusCreator  Inputs=3
  Bus Creator1 : BusCreator  Inputs=3
  Bus Selector2 : BusSelector  OutputSignals=B,A
  Demux : Demux  Outputs=2
  Dot Product : DotProduct  InputSameDT=on  OutDataTypeStr=Inherit: Inherit via internal rule
  Dot Product1 : DotProduct  InputSameDT=on  OutDataTypeStr=Inherit: Inherit via internal rule
  Dot Product2 : DotProduct  InputSameDT=on  OutDataTypeStr=Inherit: Inherit via internal rule
  Mux1 : Mux  Inputs=2
  Selector : Selector  NumberOfDimensions=2  InputPortWidth=3  IndexOptions=Index vector (dialog),Index vector (dialog)  Indices=1,[1 2 3]  OutputSizes=1,1
  Selector1 : Selector  NumberOfDimensions=2  InputPortWidth=3  IndexOptions=Index vector (dialog),Index vector (dialog)  Indices=2,[1 2 3]  OutputSizes=1,1
  Selector2 : Selector  NumberOfDimensions=2  InputPortWidth=3  IndexOptions=Index vector (dialog),Index vector (dialog)  Indices=1,[2 3]  OutputSizes=1,1
  Sum : Sum  Inputs=+++-
  Unit Delay{,1..5} (6 alike) : UnitDelay  SampleTime=-1  HasFrameUpgradeWarning=on
  Model Output : Outport
  wires:
  Parameters/1 -> Bus Selector2/1
  Bus Selector2/1 -> Selector1/1, Selector/1  "<B>"
  u/1 -> Demux/1
  Demux/1 -> Unit Delay/1, Bus Creator/1
  Unit Delay/1 -> Unit Delay1/1, Bus Creator/2
  Unit Delay1/1 -> Bus Creator/3
  Bus Creator/1 -> Dot Product/1
  Selector/1 -> Dot Product/2
  Unit Delay2/1 -> Unit Delay3/1, Bus Creator1/2
  Demux/2 -> Unit Delay2/1, Bus Creator1/1
  Unit Delay3/1 -> Bus Creator1/3
  Bus Creator1/1 -> Dot Product1/1
  Selector1/1 -> Dot Product1/2
  Sum/1 -> Unit Delay4/1, Model Output/1
  Dot Product/1 -> Sum/2
  Dot Product1/1 -> Sum/3
  e/1 -> Sum/1
  Unit Delay4/1 -> Unit Delay5/1, Mux1/1
  Unit Delay5/1 -> Mux1/2
  Dot Product2/1 -> Sum/4
  Bus Selector2/2 -> Selector2/1  "<A>"
  Selector2/1 -> Dot Product2/1
  Mux1/1 -> Dot Product2/2
